simulink model "scaling_signal"  (R2021a)
settings: Solver=VariableStepAuto  StartTime=0.0  StopTime=10.0  RelTol=1e-3
settings Model: Creator=Beshary  LastModifiedBy=Beshary

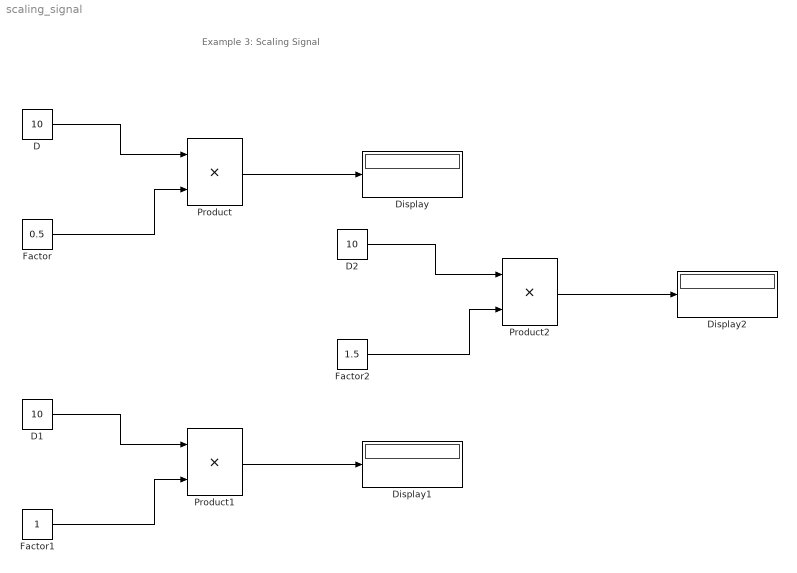
== system scaling_signal ==
  note: Example 3: Scaling Signal
  D : Constant  Value=10
  D1 : Constant  Value=10
  D2 : Constant  Value=10
  Display : Display
  Display1 : Display
  Display2 : Display
  Factor : Constant  Value=0.5
  Factor1 : Constant
  Factor2 : Constant  Value=1.5
  Product : Product
  Product1 : Product
  Product2 : Product
  wires:
  D/1 -> Product/1
  Factor/1 -> Product/2
  Product/1 -> Display/1
  Product1/1 -> Display1/1
  Factor1/1 -> Product1/2
  D1/1 -> Product1/1
  D2/1 -> Product2/1
  Factor2/1 -> Product2/2
  Product2/1 -> Display2/1
